simulink model "Simulation_Example_v3_pub"  (R2019a)
settings: Solver=VariableStepAuto  StartTime=0.0  StopTime=40  RelTol=1e-3
undefined symbols (not defined in the file or in its folder): stdval
libraries: SY202_NCS_Library x10
settings Model: Creator=rodrigue  LastModifiedBy=rodrigue
settings DataIOCC: ReturnWorkspaceOutputs=off
settings DebuggingCC: ArithmeticOperatorsInVariantConditions=warning
settings SFSimCC: SimUseLocalCustomCode=off
settings RTWCC: RTWUseLocalCustomCode=off

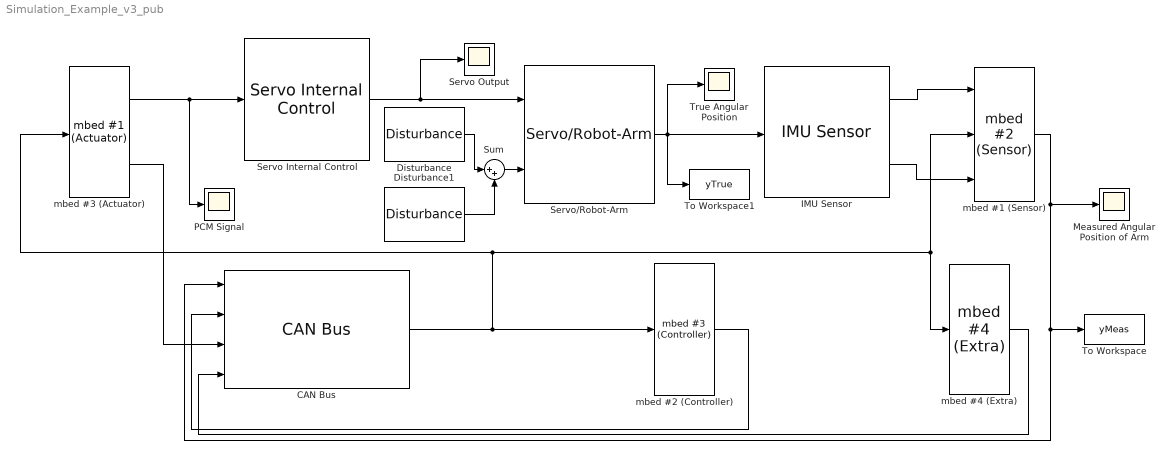
== system Simulation_Example_v3_pub ==
  CAN Bus : SY202_NCS_Library/CAN Bus
  Disturbance : SY202_NCS_Library/Disturbance  DisturbanceTime=10  DisturbanceValue=.5
  Disturbance1 : SY202_NCS_Library/Disturbance  DisturbanceTime=20  DisturbanceValue=-.5
  IMU Sensor : SY202_NCS_Library/IMU Sensor  MeanSensorError=0  MeanSensorVar=stdval^2
  Measured Angular Position of Arm : Scope
  PCM Signal : Scope
  Servo Internal Control : SY202_NCS_Library/Servo Internal Control  MaxPW=2100  MinPW=900  MaxServo=pi/3  MinServo=-pi/3
  Servo Output : Scope
  Servo/Robot-Arm : SY202_NCS_Library/Servo//Robot-Arm  x0=-.5  xdot0=0  MaxPW=2100  MinPW=900  MaxServo=pi/3  MinServo=-pi/3
  Sum : Sum  Inputs=|++
  To Workspace : ToWorkspace  VariableName=yMeas  SampleTime=-1
  To Workspace1 : ToWorkspace  VariableName=yTrue  SampleTime=-1
  True Angular Position : Scope
  mbed #1 (Sensor) : SY202_NCS_Library/mbed #2 (Sensor)
  mbed #2 (Controller) : SY202_NCS_Library/mbed #3 (Controller)  DesValue=0  Kp=100  Ki=500  Offset=1600
  mbed #3 (Actuator) : SY202_NCS_Library/mbed #1 (Actuator)  MinPW=900  MaxPW=2100
  mbed #4 (Extra) : SY202_NCS_Library/mbed #4 (Extra)  AttackRate=50  AttackMode=Replay Attack (Variant)  AttackMag=0  AttackTime=50
  wires:
  mbed #1 (Sensor)/1 -> Measured Angular Position of Arm/1, To Workspace/1, CAN Bus/1
  mbed #3 (Actuator)/1 -> Servo Internal Control/1, PCM Signal/1
  Servo Internal Control/1 -> Servo Output/1, Servo/Robot-Arm/1
  Servo/Robot-Arm/1 -> To Workspace1/1, IMU Sensor/1, True Angular Position/1
  IMU Sensor/1 -> mbed #1 (Sensor)/1
  IMU Sensor/2 -> mbed #1 (Sensor)/3
  mbed #3 (Actuator)/2 -> CAN Bus/3
  mbed #2 (Controller)/1 -> CAN Bus/2
  mbed #4 (Extra)/1 -> CAN Bus/4
  CAN Bus/1 -> mbed #4 (Extra)/1, mbed #1 (Sensor)/2, mbed #3 (Actuator)/1, mbed #2 (Controller)/1
  Sum/1 -> Servo/Robot-Arm/2
  Disturbance/1 -> Sum/1
  Disturbance1/1 -> Sum/2
